simulink model "Charging_Circuit_01"  (R2017a)
settings: Solver=VariableStepAuto  StartTime=0.0  StopTime=10.0  MaxStep=1e-4  RelTol=1e-3
libraries: powerlib x5
settings Model: Creator=judithlopez  LastModifiedBy=judithlopez
settings DebuggingCC: AlgebraicLoopMsg=none

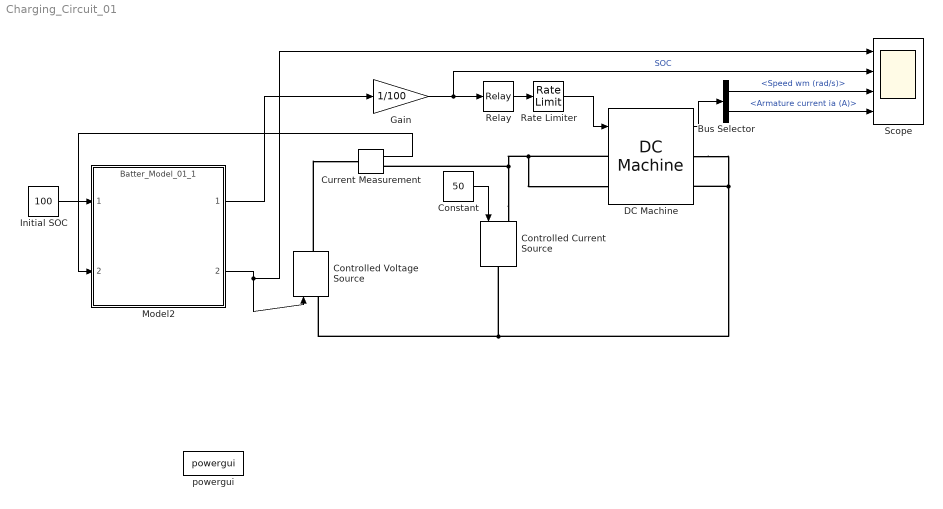
== system Charging_Circuit_01 ==
  Bus Selector : BusSelector  OutputSignals=Speed wm (rad/s),Armature current ia (A)
  Constant : Constant  Value=50
  Controlled Current Source : powerlib/Electrical Sources/Controlled Current Source  Initialize=on  Source_Type=AC  Amplitude=0  Phase=0  Frequency=0  Measurements=None
  Controlled Voltage Source : powerlib/Electrical Sources/Controlled Voltage Source  Initialize=on  Source_Type=AC  Amplitude=0  Phase=0  Frequency=0  Measurements=None
  Current Measurement : powerlib/Measurements/Current Measurement  PhasorSimulation=off  OutputType=Complex  PSBequivalent=0
  DC Machine : powerlib/Machines/DC Machine  PresetModel=No  MechanicalLoad=Torque TL  FieldType=Wound  ShowDetailedParameters=on  MeasurementBus=off  RLa=[0.4832 0.006763]  RLf=[84.91 13.39]  Laf=0.7096  MachineConstant=Torque constant (N.m/A)  Ke=1.8  Kt=1.8  J=0.2053  Bm=0.007032  Tf=0  w0=0  Ifinit=0  TsPowergui=0  TsBlock=-1
  Gain : Gain  Gain=1/100
  Initial SOC : Constant  Value=100
  Model2 : ModelReference  ModelNameDialog=Batter_Model_01_1.mdl  SimulationMode=Normal  ModelReferenceVersion=1.8
  Rate Limiter : RateLimiter  RisingSlewLimit=100  FallingSlewLimit=-100
  Relay : Relay  OnSwitchValue=0.8  OffSwitchValue=0.4  OnOutputValue=0  OffOutputValue=-200
  Scope : Scope  NumInputPorts=4
  powergui : powerlib/powergui  SimulationMode=Continuous  SampleTime=0.001  frequency=60  Iterations=50  frequencyindice=0  Pbase=100e6  ErrMax=1e-4  UnitsV=kV  UnitsW=MW  buscounter=0  FunctionMessages=off  echomessages=off  EnableUseOfTLC=off  CurrentSourceSwitches=off  DisableSnubberDevices=off  DisableRonSwitches=off  DisableVfSwitches=off  DisplayEquations=off  SolverType=Tustin/Backward Euler (TBE)  Interpol=off  ExternalGateDelay=off  methode=off  Ts=100  x0status=blocks  SPID=on  SwTol=0  HookPort=off  RestoreLinks=warning  ResistiveCurrentMeasurement=off  Frange=[0:2:500]  Ylog=off  Xlog=on  ShowGrid=off  save=off  variable=ZData  structure=0  ZoomFFT=on  StartTime=0.0  cycles=1  DisplayStyle=1  fundamental=60  FreqAxis=off  MaxFrequency=1000  frequencyindicesteady=1  RmsSteady=1  display=off
  wires:
  Relay/1 -> Rate Limiter/1
  Bus Selector/1 -> Scope/3  "<Speed wm (rad/s)>"
  DC Machine/1 -> Bus Selector/1
  Rate Limiter/1 -> DC Machine/1
  Gain/1 -> Relay/1, Scope/2  "SOC"
  Constant/1 -> Controlled Current Source/1
  Bus Selector/2 -> Scope/4  "<Armature current ia (A)>"
  Initial SOC/1 -> Model2/1
  Current Measurement/1 -> Model2/2
  Model2/1 -> Gain/1
  Model2/2 -> Scope/1, Controlled Voltage Source/1
  connections:
  Controlled Current Source/LConn1 -- DC Machine/LConn1 -- DC Machine/LConn2 -- Current Measurement/RConn1
  DC Machine/RConn2 -- Controlled Voltage Source/LConn1 -- Controlled Current Source/RConn1 -- DC Machine/RConn1
  Controlled Voltage Source/RConn1 -- Current Measurement/LConn1
